simulink model "kurvenradius_modification"  (R2020a)
settings: Solver=VariableStepAuto  StartTime=0.0  StopTime=1  RelTol=1e-3
settings Model: Creator=Besitzer  LastModifiedBy=Besitzer

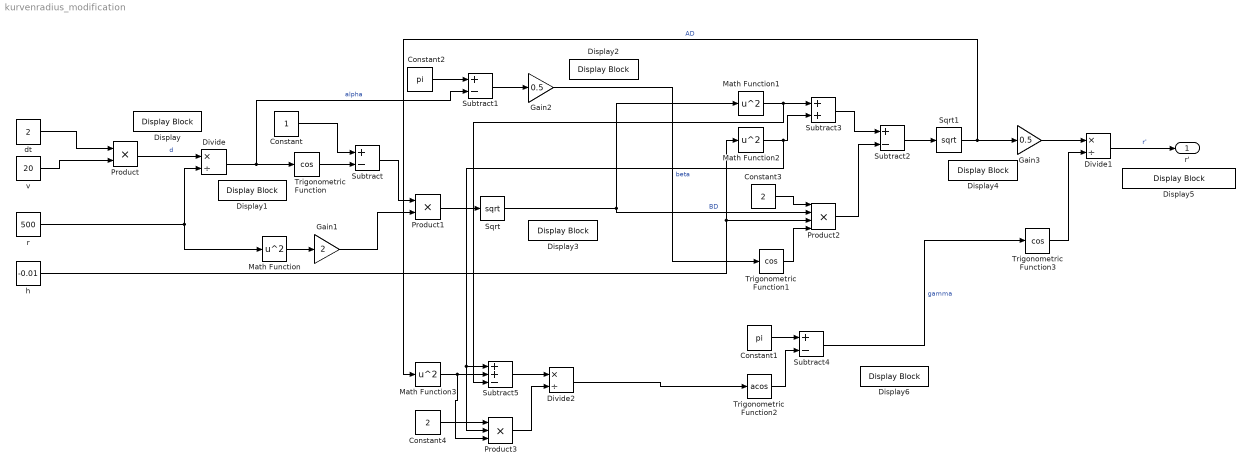
== system kurvenradius_modification ==
  Constant : Constant
  Constant1 : Constant  Value=pi
  Constant2 : Constant  Value=pi
  Constant3 : Constant  Value=2
  Constant4 : Constant  Value=2
  Display{,1..6} (7 alike) : DisplayBlock  LabelPosition=Hide  Format=short  Transparency=1
  Divide : Product  Inputs=*/
  Divide1 : Product  Inputs=*/
  Divide2 : Product  Inputs=*/
  Gain1 : Gain  Gain=2
  Gain2 : Gain  Gain=0.5
  Gain3 : Gain  Gain=0.5
  Math Function{,1..3} (4 alike) : Math  Operator=square  SaturateOnIntegerOverflow=on
  Product : Product
  Product1 : Product
  Product2 : Product  Inputs=4
  Product3 : Product  Inputs=3
  Sqrt : Sqrt  SaturateOnIntegerOverflow=on
  Sqrt1 : Sqrt  SaturateOnIntegerOverflow=on
  Subtract{,1..2,4} (4 alike) : Sum  Inputs=+-
  Subtract3 : Sum
  Subtract5 : Sum  Inputs=++-
  Trigonometric Function : Trigonometry  Operator=cos
  Trigonometric Function1 : Trigonometry  Operator=cos
  Trigonometric Function2 : Trigonometry  Operator=acos
  Trigonometric Function3 : Trigonometry  Operator=cos
  dt : Constant  Value=2
  h : Constant  Value=-0.01
  r : Constant  Value=500
  v : Constant  Value=20
  r' : Outport
  wires:
  dt/1 -> Product/1
  v/1 -> Product/2
  Product/1 -> Divide/1  "d"
  r/1 -> Math Function/1, Divide/2
  Divide/1 -> Subtract1/2, Trigonometric Function/1  "alpha"
  Math Function/1 -> Gain1/1
  Constant/1 -> Subtract/1
  Trigonometric Function/1 -> Subtract/2
  Subtract/1 -> Product1/1
  Gain1/1 -> Product1/2
  Product1/1 -> Sqrt/1
  Sqrt/1 -> Math Function1/1, Product2/2  "BD"
  Constant2/1 -> Subtract1/1
  Subtract1/1 -> Gain2/1
  Gain2/1 -> Trigonometric Function1/1  "beta"
  Subtract2/1 -> Sqrt1/1
  Subtract3/1 -> Subtract2/1
  h/1 -> Product2/3, Math Function2/1
  Math Function2/1 -> Product3/2, Subtract5/1, Subtract3/2
  Product2/1 -> Subtract2/2
  Constant3/1 -> Product2/1
  Sqrt1/1 -> Math Function3/1, Gain3/1  "AD"
  Gain3/1 -> Divide1/1
  Trigonometric Function1/1 -> Product2/4
  Divide1/1 -> r'/1  "r'"
  Constant1/1 -> Subtract4/1
  Trigonometric Function2/1 -> Subtract4/2
  Math Function3/1 -> Product3/3, Subtract5/2
  Math Function1/1 -> Subtract5/3, Subtract3/1
  Subtract5/1 -> Divide2/1
  Constant4/1 -> Product3/1
  Product3/1 -> Divide2/2
  Divide2/1 -> Trigonometric Function2/1
  Subtract4/1 -> Trigonometric Function3/1  "gamma"
  Trigonometric Function3/1 -> Divide1/2
